simulink model "sampleModel1444_1_sub_sub"  (R2023a)
settings: Solver=VariableStepAuto  StartTime=0.0  StopTime=10.0  RelTol=1e-3
libraries: hdlsllib x2, simulink x2
settings Model: Creator=user1  LastModifiedBy=user1
settings OptimizationCC: BlockReduction=off  ConditionallyExecuteInputs=off

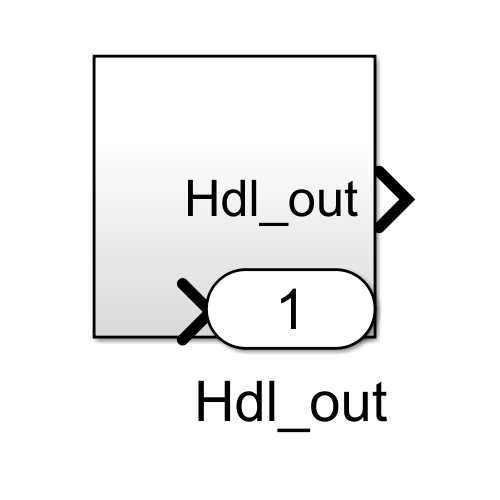
[thumbnail: Simulink's stored preview of the top-level diagram]
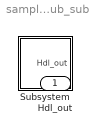
== system sampleModel1444_1_sub_sub ==
  Subsystem : Subsystem
  Hdl_out : Outport  OutDataTypeStr=uint8

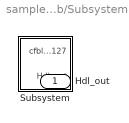
== system sampleModel1444_1_sub_sub/Subsystem ==
  Subsystem : Subsystem
  Hdl_out : Outport  OutDataTypeStr=uint8

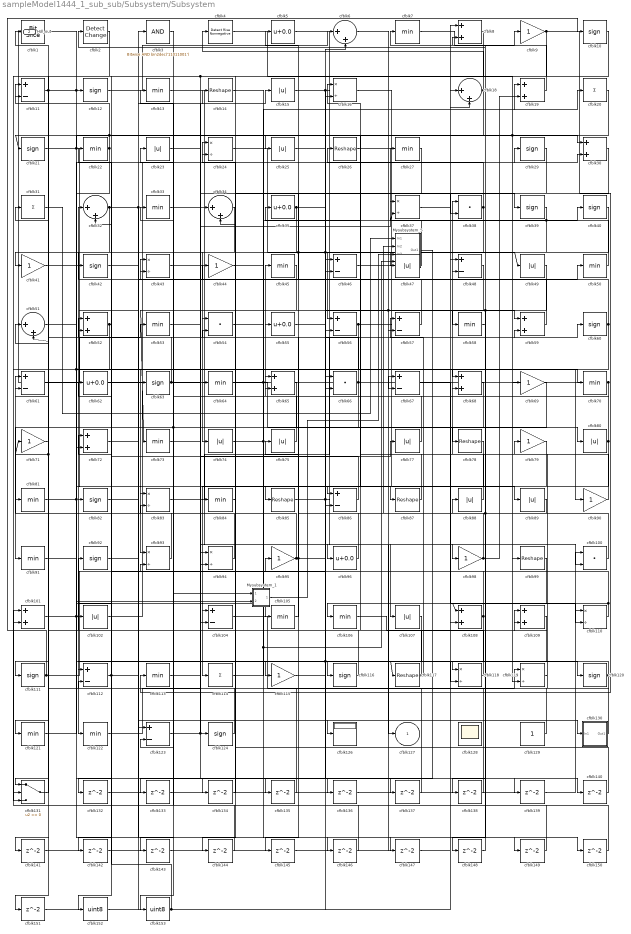
== system sampleModel1444_1_sub_sub/Subsystem/Subsystem ==
  Mysubsystem_1 : Subsystem  TreatAsAtomicUnit=on  RTWFcnName=Mysubsystem_1
      settings: RTWFcnNameOpts=User specified  RTWFileNameOpts=Use function name
  Mysubsystem_5 : Subsystem  TreatAsAtomicUnit=on  RTWFcnName=Mysubsystem_5
      settings: RTWFcnNameOpts=User specified  RTWFileNameOpts=Use function name
  cfblk1 : hdlsllib/Logic and Bit Operations/Bit Slice  lidx=7  ridx=0
  cfblk{10,12,21,29,39..40,42,60,63,82,92,111,116,120,124} (15 alike) : Signum
  cfblk{38,54,66,100} (4 alike) : DotProduct  OutDataTypeStr=uint8
  cfblk{8,19,30,52,59,65,68,72,101,108..109} (11 alike) : Sum  OutDataTypeStr=uint8
  cfblk{15,23,25,47,49,74..75,77,80,88..89,102,107} (13 alike) : Abs  OutDataTypeStr=uint8  SaturateOnIntegerOverflow=off
  cfblk{11,46,48,56..57,61,67,86,104,112,123} (11 alike) : Sum  Inputs=+-  OutDataTypeStr=uint8
  cfblk{7,13,22,27,33,45,50,53,58,64,70,73,81,84,91,105..106,113,121..122} (20 alike) : MinMax  OutDataTypeStr=uint8
  cfblk{16,24,37,43,83,93..94,110,118..119} (10 alike) : Product  Inputs=*/  OutDataTypeStr=uint8  RndMeth=Zero  SaturateOnIntegerOverflow=on
  cfblk114 : Sum  Inputs=+  OutDataTypeStr=uint8
  cfblk{9,41,44,69,71,79,90,95,98,115} (10 alike) : Gain  OutDataTypeStr=uint8
  cfblk{14,26,78,85,87,99,117} (7 alike) : Reshape
  cfblk126 : Display
  cfblk128 : Scope
      settings: Floating=on
  cfblk129 : Constant  OutDataTypeStr=uint8  SampleTime=-1
  cfblk130 : Subsystem
      settings: LibrarySourceBlock=|
      | hdlsllib/Ports &
      | Subsystems/Subsystem
  cfblk131 : Switch  OutDataTypeStr=uint8  SaturateOnIntegerOverflow=off  InputSameDT=off
  cfblk{132..151} (20 alike) : Delay  SampleTime=1
  cfblk152 : DataTypeConversion  OutDataTypeStr=uint8  SaturateOnIntegerOverflow=off  RndMeth=Floor
  cfblk153 : DataTypeConversion  OutDataTypeStr=uint8  SaturateOnIntegerOverflow=off  RndMeth=Floor
  cfblk{6,18,32,34,51} (5 alike) : Sum  Inputs=|++  OutDataTypeStr=uint8
  cfblk2 : simulink/Logic and Bit Operations/Detect Change  vinit=0  OutDataTypeStr=uint8
      settings: LibrarySourceBlock=|
      | hdlsllib/Logic and Bit
      | Operations/Detect
      | Change
  cfblk20 : Sum  Inputs=+  OutDataTypeStr=uint8
  cfblk3 : simulink/Logic and Bit Operations/Bitwise Operator  logicop=AND  UseBitMask=on  BitMask=bin2dec('11011001')  BitMaskRealWorld=Stored Integer
      settings: LibrarySourceBlock=|
      | hdlsllib/Logic and Bit
      | Operations/Bitwise
      | Operator
  cfblk31 : Sum  Inputs=+  OutDataTypeStr=uint8
  cfblk{5,35,55,62,96} (5 alike) : Bias  Bias=0.0  SaturateOnIntegerOverflow=off
  cfblk4 : hdlsllib/Logic and Bit Operations/Detect Rise Nonnegative  vinit=0  OutDataTypeStr=uint8
  cfblk127 : Outport  OutDataTypeStr=uint8  VectorParamsAs1DForOutWhenUnconnected=off
  Hdl_out : Outport  Port=2  OutDataTypeStr=uint8
  wires:
  Mysubsystem_5/1(Out1) -> cfblk133/1
  Mysubsystem_1/1(Out1) -> Mysubsystem_5/3(In3)
  cfblk31/1 -> Mysubsystem_5/1(In1)
  cfblk153/1 -> cfblk52/2, cfblk18/2
  cfblk152/1 -> cfblk3/1
  cfblk107/1 -> cfblk152/1
  cfblk151/1 -> cfblk56/2
  cfblk150/1 -> cfblk131/2
  cfblk149/1 -> cfblk83/2
  cfblk148/1 -> cfblk8/2
  cfblk147/1 -> cfblk18/1
  cfblk54/1 -> cfblk147/1
  cfblk146/1 -> cfblk101/1
  cfblk14/1 -> cfblk146/1
  cfblk145/1 -> cfblk66/1
  cfblk144/1 -> cfblk123/2
  cfblk143/1 -> cfblk46/1
  cfblk45/1 -> cfblk143/1
  cfblk142/1 -> cfblk48/1
  cfblk141/1 -> cfblk67/1
  cfblk2/1 -> cfblk141/1
  cfblk140/1 -> cfblk24/2
  cfblk139/1 -> cfblk100/1
  cfblk82/1 -> cfblk139/1
  cfblk138/1 -> cfblk51/1
  cfblk58/1 -> cfblk138/1
  cfblk137/1 -> cfblk93/2
  cfblk136/1 -> cfblk108/2
  cfblk53/1 -> cfblk136/1
  cfblk135/1 -> cfblk1/1
  cfblk79/1 -> cfblk135/1
  cfblk134/1 -> cfblk34/2
  cfblk109/1 -> cfblk134/1
  cfblk133/1 -> cfblk6/2
  cfblk132/1 -> cfblk110/1
  cfblk77/1 -> cfblk33/1
  cfblk99/1 -> cfblk106/1
  cfblk23/1 -> cfblk39/1
  cfblk67/1 -> cfblk110/2
  cfblk37/1 -> cfblk20/1
  cfblk60/1 -> cfblk5/1, cfblk131/3
  cfblk49/1 -> cfblk104/2, cfblk148/1
  cfblk86/1 -> cfblk42/1
  cfblk4/1 -> cfblk99/1
  cfblk20/1 -> cfblk86/1, cfblk119/2
  cfblk87/1 -> cfblk35/1
  cfblk123/1 -> cfblk124/1, cfblk77/1
  cfblk11/1 -> cfblk30/1, cfblk151/1
  cfblk83/1 -> cfblk8/1
  cfblk38/1 -> cfblk142/1, cfblk145/1, cfblk16/1
  cfblk84/1 -> cfblk54/2
  cfblk8/1 -> cfblk94/2, cfblk102/1
  cfblk71/1 -> cfblk11/1
  cfblk96/1 -> cfblk65/1
  cfblk112/1 -> cfblk72/1, cfblk149/1
  cfblk70/1 -> cfblk68/2, Hdl_out/1
  cfblk63/1 -> cfblk31/1, cfblk37/1
  cfblk57/1 -> cfblk32/1
  cfblk25/1 -> cfblk38/2
  cfblk81/1 -> cfblk83/1, cfblk104/1
  cfblk101/1 -> Mysubsystem_1/2(In2), cfblk105/1, cfblk150/1
  cfblk91/1 -> cfblk118/2
  cfblk51/1 -> cfblk66/2, cfblk137/1
  cfblk117/1 -> cfblk92/1, cfblk57/1
  cfblk39/1 -> cfblk47/1, cfblk37/2
  cfblk124/1 -> cfblk13/1
  cfblk29/1 -> cfblk54/1
  cfblk33/1 -> cfblk100/2
  cfblk100/1 -> Mysubsystem_5/2(In2), cfblk48/2
  cfblk42/1 -> cfblk130/1(In1)
  cfblk52/1 -> cfblk121/1, cfblk32/2
  cfblk47/1 -> cfblk27/1
  cfblk15/1 -> cfblk69/1, cfblk59/1
  cfblk18/1 -> cfblk131/1, cfblk4/1
  cfblk59/1 -> cfblk23/1
  cfblk61/1 -> cfblk53/1
  cfblk3/1 -> cfblk153/1
  cfblk21/1 -> cfblk123/1, cfblk25/1
  cfblk75/1 -> cfblk43/2
  cfblk121/1 -> cfblk29/1
  cfblk72/1 -> cfblk118/1
  cfblk113/1 -> cfblk94/1
  cfblk6/1 -> cfblk67/2
  cfblk118/1 -> cfblk26/1
  cfblk108/1 -> cfblk95/1, cfblk132/1
  cfblk1/1 -> cfblk12/1, cfblk86/2
  cfblk30/1 -> cfblk115/1
  cfblk26/1 -> cfblk58/1
  cfblk85/1 -> cfblk127/1, cfblk59/2
  cfblk129/1 -> cfblk52/1
  cfblk27/1 -> cfblk46/2
  cfblk22/1 -> cfblk21/1, cfblk11/2, cfblk72/2
  cfblk131/1 -> cfblk81/1
  cfblk34/1 -> cfblk63/1
  cfblk90/1 -> cfblk43/1
  cfblk19/1 -> cfblk7/1
  cfblk48/1 -> cfblk73/1, cfblk57/2
  cfblk119/1 -> cfblk79/1
  cfblk44/1 -> cfblk68/1
  cfblk93/1 -> cfblk51/2, cfblk71/1
  cfblk98/1 -> cfblk55/1, cfblk19/2
  cfblk78/1 -> cfblk114/1
  cfblk73/1 -> cfblk15/1
  cfblk95/1 -> cfblk60/1, cfblk65/2, cfblk44/1
  cfblk10/1 -> cfblk101/2
  cfblk69/1 -> cfblk111/1
  cfblk115/1 -> cfblk120/1
  cfblk16/1 -> cfblk80/1
  cfblk116/1 -> cfblk61/2
  cfblk7/1 -> cfblk9/1
  cfblk110/1 -> cfblk108/1, cfblk62/1
  cfblk66/1 -> Mysubsystem_1/1(In1), cfblk112/1, cfblk22/1
  cfblk35/1 -> cfblk98/1, cfblk49/1, cfblk82/1
  cfblk43/1 -> cfblk64/1
  cfblk92/1 -> cfblk50/1
  cfblk46/1 -> cfblk89/1
  cfblk122/1 -> cfblk34/1
  cfblk74/1 -> cfblk87/1, cfblk19/1
  cfblk55/1 -> cfblk117/1, cfblk140/1
  cfblk111/1 -> cfblk10/1, cfblk16/2
  cfblk12/1 -> cfblk6/1
  cfblk64/1 -> cfblk78/1, cfblk30/2
  cfblk114/1 -> Mysubsystem_5/4(In4), cfblk40/1
  cfblk65/1 -> cfblk91/1
  cfblk94/1 -> cfblk61/1
  cfblk24/1 -> cfblk56/1
  cfblk32/1 -> cfblk126/1, cfblk14/1, cfblk41/1
  cfblk130/1(Out1) -> cfblk109/2
  cfblk9/1 -> cfblk113/1, cfblk84/1
  cfblk68/1 -> cfblk122/1
  cfblk40/1 -> cfblk74/1
  cfblk106/1 -> cfblk109/1
  cfblk56/1 -> cfblk93/1, cfblk90/1
  cfblk62/1 -> cfblk70/1
  cfblk5/1 -> cfblk107/1
  cfblk89/1 -> cfblk88/1
  cfblk102/1 -> cfblk24/1
  cfblk105/1 -> cfblk75/1
  cfblk80/1 -> cfblk45/1, cfblk144/1
  cfblk104/1 -> cfblk119/1
  cfblk41/1 -> cfblk85/1
  cfblk50/1 -> cfblk2/1
  cfblk120/1 -> cfblk116/1, cfblk112/2
  cfblk88/1 -> cfblk38/1
  cfblk13/1 -> cfblk96/1

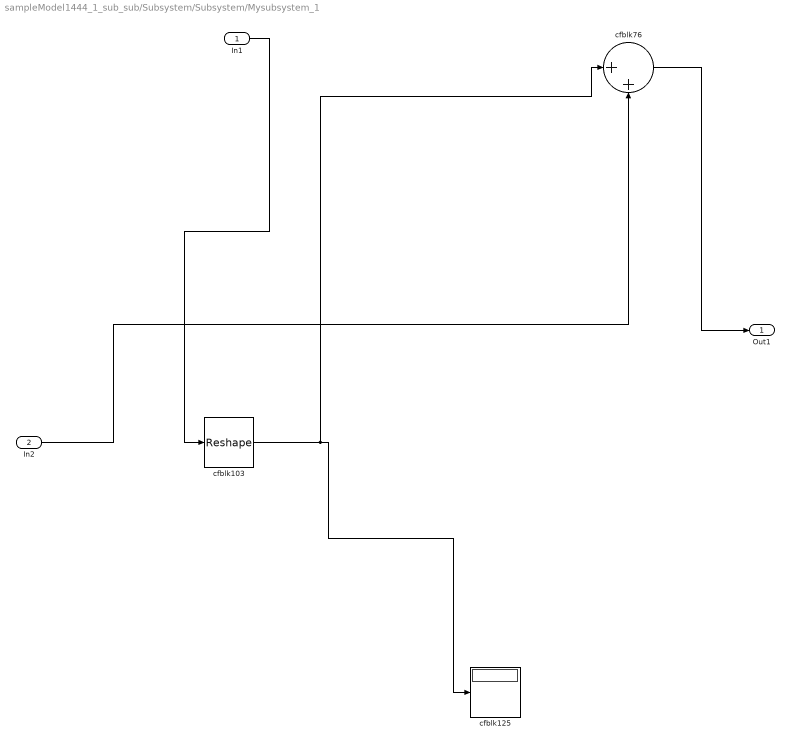
== system sampleModel1444_1_sub_sub/Subsystem/Subsystem/Mysubsystem_1 ==
  In1 : Inport
  In2 : Inport  Port=2
  cfblk103 : Reshape
  cfblk125 : Display
  cfblk76 : Sum  Inputs=|++
  Out1 : Outport
  wires:
  cfblk103/1 -> cfblk125/1, cfblk76/1
  cfblk76/1 -> Out1/1
  In1/1 -> cfblk103/1
  In2/1 -> cfblk76/2

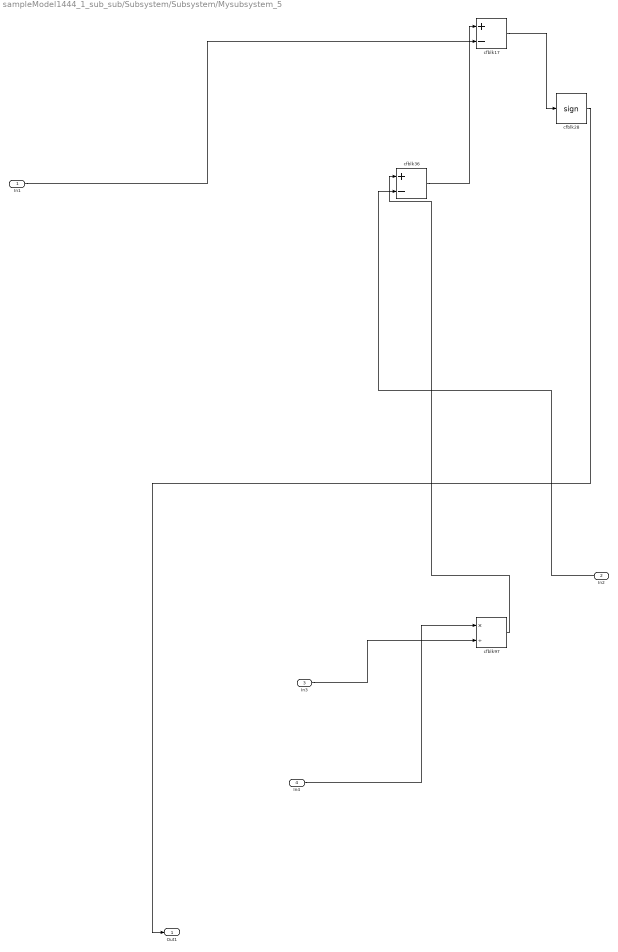
== system sampleModel1444_1_sub_sub/Subsystem/Subsystem/Mysubsystem_5 ==
  In1 : Inport
  In2 : Inport  Port=2
  In3 : Inport  Port=3
  In4 : Inport  Port=4
  cfblk17 : Sum  Inputs=+-
  cfblk28 : Signum
  cfblk36 : Sum  Inputs=+-
  cfblk97 : Product  Inputs=*/  RndMeth=Zero  SaturateOnIntegerOverflow=on
  Out1 : Outport
  wires:
  cfblk36/1 -> cfblk17/1
  In1/1 -> cfblk17/2
  cfblk28/1 -> Out1/1
  In4/1 -> cfblk97/1
  cfblk17/1 -> cfblk28/1
  cfblk97/1 -> cfblk36/1
  In3/1 -> cfblk97/2
  In2/1 -> cfblk36/2

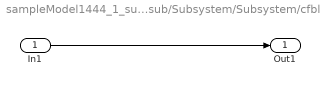
== system sampleModel1444_1_sub_sub/Subsystem/Subsystem/cfblk130 ==
  In1 : Inport
  Out1 : Outport
  wires:
  In1/1 -> Out1/1
